simulink model "mariner_simtr"  (R2018b)
settings: Solver=FixedStepAuto  StartTime=0.0  StopTime=600  FixedStep=0.1  RelTol=1e-3
libraries: neural x211, simulink x2
(part 2 of 10)

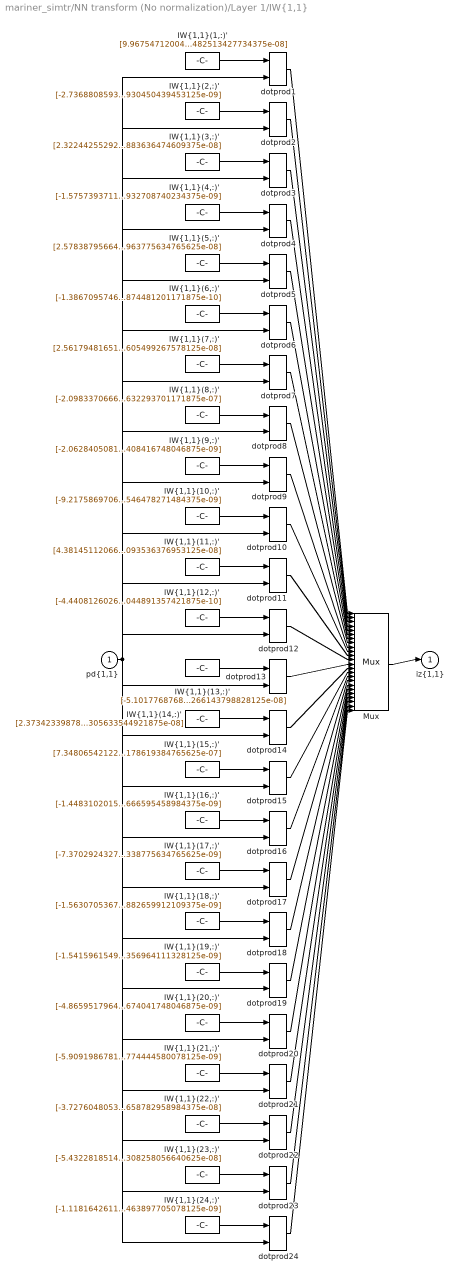
== system mariner_simtr/NN transform (No normalization)/Layer 1/IW{1,1} ==
  "pd{1,1}" : Inport  PortDimensions=7
      mask Display: e = 0.06;c1 = [120 230 180]/255;c2 = ([120 230 180]+0)/(256+128);c3 = ([120 230 180]+128)/(256+128);patch([0 1 1 0],[0 0 1 1],c1);patch([0 1 1 1-e 1-e 0+e],[0 0 1 1-e 0+e 0+e],c2);patch([0 0 1 1-e 0+e 0+e],[0 1 1 1-e 1-e 0+e],c3);plot([0 1 1 0 0],[0 0 1 1 0]);
  "IW{1,1}(1,:)'" : Constant  Value=[9.96754712004838051999594400747091438308444821814191527664661407470703125e-10;-4.23539616837629799060249528863675294587665121071040630340576171875e-08;1.955485657944718495509006986853017817651334553374908864498138427734375e-08;-4.070098816021972745819758874620541977407128797494806349277496337890625e-08;4.66661762648838560338676137331619109271940715188975445926189422607421875e-09;-4.813604277413395185011998032853508533435160643421113491058349609375e-08;-3.648399644882457702946610181814202089611853807582519948482513427734375e-08]
      mask Display: e = 0.06;c1 = [120 150 230]/255;c2 = ([120 150 230]+0)/383;c3 = ([120 150 230]+128)/383;patch([0 1 1 0],[0 0 1 1],c1);patch([0 1 1 1-e 1-e 0+e],[0 0 1 1-e 0+e 0+e],c2);patch([0 0 1 1-e 0+e 0+e],[0 1 1 1-e 1-e 0+e],c3);plot([0 1 1 0 0],[0 0 1 1 0]);disp('Weights');
  "IW{1,1}(10,:)'" : Constant  Value=[-9.21758697067975692512585843448047473458473177743144333362579345703125e-09;1.5109007388292643668241629927896652052510262365103699266910552978515625e-08;-2.8593879081023034796134684831607486454885247439960949122905731201171875e-08;7.24476771790234500451820988799027378757244832740980200469493865966796875e-09;-2.390110051996968584293398892536008926157364840037189424037933349609375e-08;1.2024606259677698783971109926433686043711901447750278748571872711181640625e-09;-6.3639012808772434761134367798250666137249709208845160901546478271484375e-09]
      mask Display: e = 0.06;c1 = [120 150 230]/255;c2 = ([120 150 230]+0)/383;c3 = ([120 150 230]+128)/383;patch([0 1 1 0],[0 0 1 1],c1);patch([0 1 1 1-e 1-e 0+e],[0 0 1 1-e 0+e 0+e],c2);patch([0 0 1 1-e 0+e 0+e],[0 1 1 1-e 1-e 0+e],c3);plot([0 1 1 0 0],[0 0 1 1 0]);disp('Weights');
  "IW{1,1}(11,:)'" : Constant  Value=[4.38145112066941093156313009928108821722236854157017660327255725860595703125e-10;-2.3609184555780799633161487374559406315910337070818059146404266357421875e-08;1.08683559136344472219348574111054406277077077902504242956638336181640625e-08;-2.2688420071581493037842736592256398520106586147448979318141937255859375e-08;2.577333665822960669212732294909400099225393887536483816802501678466796875e-09;-2.6827945833227834960700084582750635231462865704088471829891204833984375e-08;-2.0338792630435224968121508200454006232149595234659500420093536376953125e-08]
      mask Display: e = 0.06;c1 = [120 150 230]/255;c2 = ([120 150 230]+0)/383;c3 = ([120 150 230]+128)/383;patch([0 1 1 0],[0 0 1 1],c1);patch([0 1 1 1-e 1-e 0+e],[0 0 1 1-e 0+e 0+e],c2);patch([0 0 1 1-e 0+e 0+e],[0 1 1 1-e 1-e 0+e],c3);plot([0 1 1 0 0],[0 0 1 1 0]);disp('Weights');
  "IW{1,1}(12,:)'" : Constant  Value=[-4.44081260262457014744597405086871944046578164488892070949077606201171875e-09;3.18447157678982755093461472391258570979744035867042839527130126953125e-08;-3.32801187487933600657970581969402612543262875988148152828216552734375e-08;2.014363404465310276539939909716536714512358230422250926494598388671875e-08;-2.7009658392937414758657856746378034262789924468961544334888458251953125e-08;1.04114761496777040929841848184052299775004257753607816994190216064453125e-08;-8.5873020309611764853519627507631717389102732340688817203044891357421875e-10]
      mask Display: e = 0.06;c1 = [120 150 230]/255;c2 = ([120 150 230]+0)/383;c3 = ([120 150 230]+128)/383;patch([0 1 1 0],[0 0 1 1],c1);patch([0 1 1 1-e 1-e 0+e],[0 0 1 1-e 0+e 0+e],c2);patch([0 0 1 1-e 0+e 0+e],[0 1 1 1-e 1-e 0+e],c3);plot([0 1 1 0 0],[0 0 1 1 0]);disp('Weights');
  "IW{1,1}(13,:)'" : Constant  Value=[-5.1017768768232909158035349832249760737568067270331084728240966796875e-09;1.099732326060325747775131880433485687120764850988052785396575927734375e-07;-9.6376903694374034393577859759771886416501729399897158145904541015625e-08;7.702898533754286069518703826408678736470392323099076747894287109375e-08;-7.235783348817856666161077612564600514133417163975536823272705078125e-08;5.267928186779311432795554876427901458413316504447720944881439208984375e-08;1.7345726966175917324916222928173070716439951866050250828266143798828125e-08]
      mask Display: e = 0.06;c1 = [120 150 230]/255;c2 = ([120 150 230]+0)/383;c3 = ([120 150 230]+128)/383;patch([0 1 1 0],[0 0 1 1],c1);patch([0 1 1 1-e 1-e 0+e],[0 0 1 1-e 0+e 0+e],c2);patch([0 0 1 1-e 0+e 0+e],[0 1 1 1-e 1-e 0+e],c3);plot([0 1 1 0 0],[0 0 1 1 0]);disp('Weights');
  "IW{1,1}(14,:)'" : Constant  Value=[2.37342339878500993051951858492203129014086471215705387294292449951171875e-09;-6.9409118276585255820877663930634771105587788042612373828887939453125e-08;3.232449834280652108462386488431372644214434330933727324008941650390625e-08;-6.66896830743175840225939860449189122704183319001458585262298583984375e-08;7.8615207967289628717666078220292769085375539361848495900630950927734375e-09;-7.8902832936415914953927710530356964824250098899938166141510009765625e-08;-5.975529031343248632389994305647018535410097683779895305633544921875e-08]
      mask Display: e = 0.06;c1 = [120 150 230]/255;c2 = ([120 150 230]+0)/383;c3 = ([120 150 230]+128)/383;patch([0 1 1 0],[0 0 1 1],c1);patch([0 1 1 1-e 1-e 0+e],[0 0 1 1-e 0+e 0+e],c2);patch([0 0 1 1-e 0+e 0+e],[0 1 1 1-e 1-e 0+e],c3);plot([0 1 1 0 0],[0 0 1 1 0]);disp('Weights');
  "IW{1,1}(15,:)'" : Constant  Value=[7.3480654212243858235158316407308054518665585419512353837490081787109375e-09;-1.37910872201280553869879772453665989218052345677278935909271240234375e-07;6.6144410053191093139834965709822345303336987853981554508209228515625e-08;-1.3245204146490021739396747597894421488717853208072483539581298828125e-07;1.708616089860501443057811429664105684622654734994284808635711669921875e-08;-1.56945855317767068446145844844152872354925420950166881084442138671875e-07;-1.18534841031160093440845193502042320687905885279178619384765625e-07]
      mask Display: e = 0.06;c1 = [120 150 230]/255;c2 = ([120 150 230]+0)/383;c3 = ([120 150 230]+128)/383;patch([0 1 1 0],[0 0 1 1],c1);patch([0 1 1 1-e 1-e 0+e],[0 0 1 1-e 0+e 0+e],c2);patch([0 0 1 1-e 0+e 0+e],[0 1 1 1-e 1-e 0+e],c3);plot([0 1 1 0 0],[0 0 1 1 0]);disp('Weights');
  "IW{1,1}(16,:)'" : Constant  Value=[-1.4483102015300659619008766631326722007511165202231495641171932220458984375e-09;3.053887482089307960456361803851244030028055931325070559978485107421875e-08;-2.68218652011502346177757743518610400457191644818522036075592041015625e-08;2.13794257743043844947837517876665369698230279027484357357025146484375e-08;-2.014676439457038581716768858853594537094977567903697490692138671875e-08;1.460163542807002359793662449836959549287485060631297528743743896484375e-08;4.7860605580468106034501928731060560462395869762985967099666595458984375e-09]
      mask Display: e = 0.06;c1 = [120 150 230]/255;c2 = ([120 150 230]+0)/383;c3 = ([120 150 230]+128)/383;patch([0 1 1 0],[0 0 1 1],c1);patch([0 1 1 1-e 1-e 0+e],[0 0 1 1-e 0+e 0+e],c2);patch([0 0 1 1-e 0+e 0+e],[0 1 1 1-e 1-e 0+e],c3);plot([0 1 1 0 0],[0 0 1 1 0]);disp('Weights');
  "IW{1,1}(17,:)'" : Constant  Value=[-7.37029243278886431384240804387010526088630513186217285692691802978515625e-09;5.13920169010480328451178516115105399109097561449743807315826416015625e-08;-5.406989574538547646120274282367790252834538478055037558078765869140625e-08;3.244029838149221145765052523417260044169552202220074832439422607421875e-08;-4.391888903266115245392352023530435634057766947080381214618682861328125e-08;1.6673505568151500479441917755389634958618216842296533286571502685546875e-08;-1.572529870117332454563925412207615883719569183085695840418338775634765625e-09]
      mask Display: e = 0.06;c1 = [120 150 230]/255;c2 = ([120 150 230]+0)/383;c3 = ([120 150 230]+128)/383;patch([0 1 1 0],[0 0 1 1],c1);patch([0 1 1 1-e 1-e 0+e],[0 0 1 1-e 0+e 0+e],c2);patch([0 0 1 1-e 0+e 0+e],[0 1 1 1-e 1-e 0+e],c3);plot([0 1 1 0 0],[0 0 1 1 0]);disp('Weights');
  "IW{1,1}(18,:)'" : Constant  Value=[-1.5630705367480064101360989086732244945920911050052382051944732666015625e-08;1.2844123921892863398315043181596717403181173722259700298309326171875e-07;-1.30133673686686352043631186188588078067596143228001892566680908203125e-07;8.200088059824167129705668223549341888656272203661501407623291015625e-08;-1.05215545994692440098363457774699458724398937192745506763458251953125e-07;4.33666531310121004011057764537806491489391191862523555755615234375e-08;-1.28883019475470923089079378922282292929679670123732648789882659912109375e-09]
      mask Display: e = 0.06;c1 = [120 150 230]/255;c2 = ([120 150 230]+0)/383;c3 = ([120 150 230]+128)/383;patch([0 1 1 0],[0 0 1 1],c1);patch([0 1 1 1-e 1-e 0+e],[0 0 1 1-e 0+e 0+e],c2);patch([0 0 1 1-e 0+e 0+e],[0 1 1 1-e 1-e 0+e],c3);plot([0 1 1 0 0],[0 0 1 1 0]);disp('Weights');
  "IW{1,1}(19,:)'" : Constant  Value=[-1.5415961549154450456600809560921312713066555488694575615227222442626953125e-09;3.3170310091952161113895030698783816802688306779600679874420166015625e-08;-2.907377317587945963731183257432177935442041416536085307598114013671875e-08;2.3233161307144997984342005910469997065348479736712761223316192626953125e-08;-2.1829287747494461351506497641915272023283023372641764581203460693359375e-08;1.5888289744811928436986789791272867145011105094454251229763031005859375e-08;5.23023291522121942520652288118043760078990089823491871356964111328125e-09]
      mask Display: e = 0.06;c1 = [120 150 230]/255;c2 = ([120 150 230]+0)/383;c3 = ([120 150 230]+128)/383;patch([0 1 1 0],[0 0 1 1],c1);patch([0 1 1 1-e 1-e 0+e],[0 0 1 1-e 0+e 0+e],c2);patch([0 0 1 1-e 0+e 0+e],[0 1 1 1-e 1-e 0+e],c3);plot([0 1 1 0 0],[0 0 1 1 0]);disp('Weights');
  "IW{1,1}(2,:)'" : Constant  Value=[-2.736880859346069335748875792926025629636654912246740423142910003662109375e-09;5.902694971324982067598831770964540321955382751184515655040740966796875e-08;-5.1728078424699451181702843267917746317152705159969627857208251953125e-08;4.134227531808641390325789505451326011353785361279733479022979736328125e-08;-3.88368911181434744954370599269444230827730279997922480106353759765625e-08;2.827394876174494392768362098673773363799455182743258774280548095703125e-08;9.309327476142742333364672670421857691991363026318140327930450439453125e-09]
      mask Display: e = 0.06;c1 = [120 150 230]/255;c2 = ([120 150 230]+0)/383;c3 = ([120 150 230]+128)/383;patch([0 1 1 0],[0 0 1 1],c1);patch([0 1 1 1-e 1-e 0+e],[0 0 1 1-e 0+e 0+e],c2);patch([0 0 1 1-e 0+e 0+e],[0 1 1 1-e 1-e 0+e],c3);plot([0 1 1 0 0],[0 0 1 1 0]);disp('Weights');
  "IW{1,1}(20,:)'" : Constant  Value=[-4.86595179647605248405393629459493587408047687858925200998783111572265625e-09;3.26657871565783989586747465029559212013055002898909151554107666015625e-08;-3.469893074219905699171392628003818270343572294223122298717498779296875e-08;2.0560448490772478499383980519131520647846400606795214116573333740234375e-08;-2.82148079239193913611238287604543462094852657173760235309600830078125e-08;1.04905239479849043770109628362537101953222418160294182598590850830078125e-08;-1.1689321922241270052697945862167638875206421289476566016674041748046875e-09]
      mask Display: e = 0.06;c1 = [120 150 230]/255;c2 = ([120 150 230]+0)/383;c3 = ([120 150 230]+128)/383;patch([0 1 1 0],[0 0 1 1],c1);patch([0 1 1 1-e 1-e 0+e],[0 0 1 1-e 0+e 0+e],c2);patch([0 0 1 1-e 0+e 0+e],[0 1 1 1-e 1-e 0+e],c3);plot([0 1 1 0 0],[0 0 1 1 0]);disp('Weights');
  "IW{1,1}(21,:)'" : Constant  Value=[-5.90919867818142536771689580263160201933914095207001082599163055419921875e-09;4.23596922702509948620164660464115780058591553824953734874725341796875e-08;-4.427960655273123418020127391690754503628113525337539613246917724609375e-08;2.6791635390820279313359056176657713166378016467206180095672607421875e-08;-3.593839528671613701771831816782210022864774146000854671001434326171875e-08;1.38421177630135737742344206207580070699947327739209868013858795166015625e-08;-1.1607068937858028159101323080470979931533292983658611774444580078125e-09]
      mask Display: e = 0.06;c1 = [120 150 230]/255;c2 = ([120 150 230]+0)/383;c3 = ([120 150 230]+128)/383;patch([0 1 1 0],[0 0 1 1],c1);patch([0 1 1 1-e 1-e 0+e],[0 0 1 1-e 0+e 0+e],c2);patch([0 0 1 1-e 0+e 0+e],[0 1 1 1-e 1-e 0+e],c3);plot([0 1 1 0 0],[0 0 1 1 0]);disp('Weights');
  "IW{1,1}(22,:)'" : Constant  Value=[-3.727604805384169344832192877388366003543751503457315266132354736328125e-08;1.172724790951451694969578996678716276136356100323610007762908935546875e-07;-1.6014903040348191092204113532282416798580015893094241619110107421875e-07;6.73183958318854417049261255022452044016745276167057454586029052734375e-08;-1.31550756612420119907568287660748485023987086606211960315704345703125e-07;2.778369009628760810329470829806164378084076815866865217685699462890625e-08;-2.029709699747728526551498301998266438062046290724538266658782958984375e-08]
      mask Display: e = 0.06;c1 = [120 150 230]/255;c2 = ([120 150 230]+0)/383;c3 = ([120 150 230]+128)/383;patch([0 1 1 0],[0 0 1 1],c1);patch([0 1 1 1-e 1-e 0+e],[0 0 1 1-e 0+e 0+e],c2);patch([0 0 1 1-e 0+e 0+e],[0 1 1 1-e 1-e 0+e],c3);plot([0 1 1 0 0],[0 0 1 1 0]);disp('Weights');
  "IW{1,1}(23,:)'" : Constant  Value=[-5.43228185145061583705953608849741065522920280272956006228923797607421875e-09;1.170978675560962556496971101634152478965233967755921185016632080078125e-07;-1.026199558971175130461586113249372598232866948819719254970550537109375e-07;8.2020122441372280621760672107700695931953305262140929698944091796875e-08;-7.70466698024706418528796572457728597527193414862267673015594482421875e-08;5.609342392485284586896892764472377646001177708967588841915130615234375e-08;1.846762772031701079541643668348316342786574750789441168308258056640625e-08]
      mask Display: e = 0.06;c1 = [120 150 230]/255;c2 = ([120 150 230]+0)/383;c3 = ([120 150 230]+128)/383;patch([0 1 1 0],[0 0 1 1],c1);patch([0 1 1 1-e 1-e 0+e],[0 0 1 1-e 0+e 0+e],c2);patch([0 0 1 1-e 0+e 0+e],[0 1 1 1-e 1-e 0+e],c3);plot([0 1 1 0 0],[0 0 1 1 0]);disp('Weights');
  "IW{1,1}(24,:)'" : Constant  Value=[-1.11816426113187927785879471659531703142675951312412507832050323486328125e-08;9.179529262955325056978187099610000387883701478131115436553955078125e-08;-9.30252272128869384096500928793549434203669079579412937164306640625e-08;5.858745564967901846581630202932811091187659258139319717884063720703125e-08;-7.52286172919048964737097177912783507736094179563224315643310546875e-08;3.096918421804722152496116530269454347745750055764801800251007080078125e-08;-1.002465361068514032997859634324840094610209462189231999218463897705078125e-09]
      mask Display: e = 0.06;c1 = [120 150 230]/255;c2 = ([120 150 230]+0)/383;c3 = ([120 150 230]+128)/383;patch([0 1 1 0],[0 0 1 1],c1);patch([0 1 1 1-e 1-e 0+e],[0 0 1 1-e 0+e 0+e],c2);patch([0 0 1 1-e 0+e 0+e],[0 1 1 1-e 1-e 0+e],c3);plot([0 1 1 0 0],[0 0 1 1 0]);disp('Weights');
  "IW{1,1}(3,:)'" : Constant  Value=[2.3224425529203732312677545030106529555524730312754400074481964111328125e-09;-6.79293542914116131004281622096652171194364200346171855926513671875e-08;3.16325922238083046083605078153955236786032401141710579395294189453125e-08;-6.5269718938136910214959057578709700209174116025678813457489013671875e-08;7.69150849643806513870867322228697116059947802568785846233367919921875e-09;-7.72232186310361172496818655923422891618201902019791305065155029296875e-08;-5.84843975722607335487583809195688555604419889277778565883636474609375e-08]
      mask Display: e = 0.06;c1 = [120 150 230]/255;c2 = ([120 150 230]+0)/383;c3 = ([120 150 230]+128)/383;patch([0 1 1 0],[0 0 1 1],c1);patch([0 1 1 1-e 1-e 0+e],[0 0 1 1-e 0+e 0+e],c2);patch([0 0 1 1-e 0+e 0+e],[0 1 1 1-e 1-e 0+e],c3);plot([0 1 1 0 0],[0 0 1 1 0]);disp('Weights');
  "IW{1,1}(4,:)'" : Constant  Value=[-1.5757393711212239489573953290200980514867978854454122483730316162109375e-09;3.398105935002767075160871163529152649829256915836594998836517333984375e-08;-2.97794683945180708540138359886884078520097318687476217746734619140625e-08;2.380147629323289543301717867233857628406212825211696326732635498046875e-08;-2.2358315984684428928152047887090159150602630688808858394622802734375e-08;1.627722399093271681704852052972876119696366004063747823238372802734375e-08;5.3590863849978235579479203163320855107798479366465471684932708740234375e-09]
      mask Display: e = 0.06;c1 = [120 150 230]/255;c2 = ([120 150 230]+0)/383;c3 = ([120 150 230]+128)/383;patch([0 1 1 0],[0 0 1 1],c1);patch([0 1 1 1-e 1-e 0+e],[0 0 1 1-e 0+e 0+e],c2);patch([0 0 1 1-e 0+e 0+e],[0 1 1 1-e 1-e 0+e],c3);plot([0 1 1 0 0],[0 0 1 1 0]);disp('Weights');
  "IW{1,1}(5,:)'" : Constant  Value=[2.578387956646821386262262190930232008678757438246975652873516082763671875e-10;-1.39061626338902988860742851624785476616352752898819744586944580078125e-08;6.40125093731916103556093254091374777914325022720731794834136962890625e-09;-1.33639767245069021187178214828648881162820316603756509721279144287109375e-08;1.5179028736585700792937570096133824415485236158929183147847652435302734375e-09;-1.580227044658806774721533238044213209860799906891770660877227783203125e-08;-1.1980281539188823830406369443969671895189321730867959558963775634765625e-08]
      mask Display: e = 0.06;c1 = [120 150 230]/255;c2 = ([120 150 230]+0)/383;c3 = ([120 150 230]+128)/383;patch([0 1 1 0],[0 0 1 1],c1);patch([0 1 1 1-e 1-e 0+e],[0 0 1 1-e 0+e 0+e],c2);patch([0 0 1 1-e 0+e 0+e],[0 1 1 1-e 1-e 0+e],c3);plot([0 1 1 0 0],[0 0 1 1 0]);disp('Weights');
  "IW{1,1}(6,:)'" : Constant  Value=[-1.3867095746777479392709234935266750243787470253664650954306125640869140625e-09;1.14066147117358784886158936007494180131516259280033409595489501953125e-08;-1.15553235223709413058554965644635081911673069043899886310100555419921875e-08;7.279280159413825905859356051562369938068286501220427453517913818359375e-09;-9.3463069187052717682138907391749260700208878915873356163501739501953125e-09;3.8464198353759935298473327945807664907107437102240510284900665283203125e-09;-1.273779272363968995991060355698720578387916901874632458202540874481201171875e-10]
      mask Display: e = 0.06;c1 = [120 150 230]/255;c2 = ([120 150 230]+0)/383;c3 = ([120 150 230]+128)/383;patch([0 1 1 0],[0 0 1 1],c1);patch([0 1 1 1-e 1-e 0+e],[0 0 1 1-e 0+e 0+e],c2);patch([0 0 1 1-e 0+e 0+e],[0 1 1 1-e 1-e 0+e],c3);plot([0 1 1 0 0],[0 0 1 1 0]);disp('Weights');
  "IW{1,1}(7,:)'" : Constant  Value=[2.561794816514778783262103480067826966060096083310781978070735931396484375e-10;-1.380210707037911175766410685865348551004672117414884269237518310546875e-08;6.35276019390252450627447865227903633922323933802545070648193359375e-09;-1.32640168703112810743202282562878957516971922814263962209224700927734375e-08;1.5058978574009581085089311055656875748542944393193465657532215118408203125e-09;-1.5685037309467738701051155625516841940481072015245445072650909423828125e-08;-1.1891651183705094023693456359476450234780031678383238613605499267578125e-08]
      mask Display: e = 0.06;c1 = [120 150 230]/255;c2 = ([120 150 230]+0)/383;c3 = ([120 150 230]+128)/383;patch([0 1 1 0],[0 0 1 1],c1);patch([0 1 1 1-e 1-e 0+e],[0 0 1 1-e 0+e 0+e],c2);patch([0 0 1 1-e 0+e 0+e],[0 1 1 1-e 1-e 0+e],c3);plot([0 1 1 0 0],[0 0 1 1 0]);disp('Weights');
  "IW{1,1}(8,:)'" : Constant  Value=[-2.098337066680637515982030296400086266661588751958333887159824371337890625e-09;-2.012744499847773860113221526535465244478473323397338390350341796875e-07;9.13914835017614789813164230015962719022581950412131845951080322265625e-08;-1.9346416131584142649138167123490372745209242566488683223724365234375e-07;2.1007094255205750548163318321658044052213654140359722077846527099609375e-08;-2.2860633849821883474575626334079903045903847669251263141632080078125e-07;-1.7352583730535906258679135043265784332788825850002467632293701171875e-07]
      mask Display: e = 0.06;c1 = [120 150 230]/255;c2 = ([120 150 230]+0)/383;c3 = ([120 150 230]+128)/383;patch([0 1 1 0],[0 0 1 1],c1);patch([0 1 1 1-e 1-e 0+e],[0 0 1 1-e 0+e 0+e],c2);patch([0 0 1 1-e 0+e 0+e],[0 1 1 1-e 1-e 0+e],c3);plot([0 1 1 0 0],[0 0 1 1 0]);disp('Weights');
  "IW{1,1}(9,:)'" : Constant  Value=[-2.0628405081894719967934079935499569469214975470094941556453704833984375e-08;1.60728119705768779211727524149078139004132026457227766513824462890625e-07;-1.64788974609277832402074435470817892479544752859510481357574462890625e-07;1.0225529152247166173080451627430687011610643821768462657928466796875e-07;-1.33437713545835176052803123895873493864883130299858748912811279296875e-07;5.35971620388351293285411906970605588895750770461745560169219970703125e-08;-2.757314565971735213566048015225266876182530495498212985694408416748046875e-09]
      mask Display: e = 0.06;c1 = [120 150 230]/255;c2 = ([120 150 230]+0)/383;c3 = ([120 150 230]+128)/383;patch([0 1 1 0],[0 0 1 1],c1);patch([0 1 1 1-e 1-e 0+e],[0 0 1 1-e 0+e 0+e],c2);patch([0 0 1 1-e 0+e 0+e],[0 1 1 1-e 1-e 0+e],c3);plot([0 1 1 0 0],[0 0 1 1 0]);disp('Weights');
  Mux : Mux  Inputs=24
      mask Display: e = 0.06;c1 = [120 150 230]/255;c2 = ([120 150 230]+0)/383;c3 = ([120 150 230]+128)/383;patch([0 1 1 0],[0 0 1 1],c1);patch([0 1 1 1-e 1-e 0+e],[0 0 1 1-e 0+e 0+e],c2);patch([0 0 1 1-e 0+e 0+e],[0 1 1 1-e 1-e 0+e],c3);plot([0 1 1 0 0],[0 0 1 1 0]);disp('Mux');
  dotprod{1..24} (24 alike) : neural/Weight Functions/dotprod
  "iz{1,1}" : Outport
      mask Display: e = 0.06;c1 = [120 230 180]/255;c2 = ([120 230 180]+0)/(256+128);c3 = ([120 230 180]+128)/(256+128);patch([0 1 1 0],[0 0 1 1],c1);patch([0 1 1 1-e 1-e 0+e],[0 0 1 1-e 0+e 0+e],c2);patch([0 0 1 1-e 0+e 0+e],[0 1 1 1-e 1-e 0+e],c3);plot([0 1 1 0 0],[0 0 1 1 0]);
  wires:
  Mux/1 -> "iz{1,1}"/1
  dotprod24/1 -> Mux/24
  "IW{1,1}(24,:)'"/1 -> dotprod24/1
  dotprod23/1 -> Mux/23
  "IW{1,1}(23,:)'"/1 -> dotprod23/1
  dotprod22/1 -> Mux/22
  "IW{1,1}(22,:)'"/1 -> dotprod22/1
  dotprod21/1 -> Mux/21
  "IW{1,1}(21,:)'"/1 -> dotprod21/1
  dotprod20/1 -> Mux/20
  "IW{1,1}(20,:)'"/1 -> dotprod20/1
  dotprod19/1 -> Mux/19
  "IW{1,1}(19,:)'"/1 -> dotprod19/1
  dotprod18/1 -> Mux/18
  "IW{1,1}(18,:)'"/1 -> dotprod18/1
  dotprod17/1 -> Mux/17
  "IW{1,1}(17,:)'"/1 -> dotprod17/1
  dotprod16/1 -> Mux/16
  "IW{1,1}(16,:)'"/1 -> dotprod16/1
  dotprod15/1 -> Mux/15
  "IW{1,1}(15,:)'"/1 -> dotprod15/1
  dotprod14/1 -> Mux/14
  "IW{1,1}(14,:)'"/1 -> dotprod14/1
  dotprod13/1 -> Mux/13
  "IW{1,1}(13,:)'"/1 -> dotprod13/1
  dotprod12/1 -> Mux/12
  "IW{1,1}(12,:)'"/1 -> dotprod12/1
  dotprod11/1 -> Mux/11
  "IW{1,1}(11,:)'"/1 -> dotprod11/1
  dotprod10/1 -> Mux/10
  "IW{1,1}(10,:)'"/1 -> dotprod10/1
  dotprod9/1 -> Mux/9
  "IW{1,1}(9,:)'"/1 -> dotprod9/1
  dotprod8/1 -> Mux/8
  "IW{1,1}(8,:)'"/1 -> dotprod8/1
  dotprod7/1 -> Mux/7
  "IW{1,1}(7,:)'"/1 -> dotprod7/1
  dotprod6/1 -> Mux/6
  "IW{1,1}(6,:)'"/1 -> dotprod6/1
  dotprod5/1 -> Mux/5
  "IW{1,1}(5,:)'"/1 -> dotprod5/1
  dotprod4/1 -> Mux/4
  "IW{1,1}(4,:)'"/1 -> dotprod4/1
  dotprod3/1 -> Mux/3
  "IW{1,1}(3,:)'"/1 -> dotprod3/1
  dotprod2/1 -> Mux/2
  "IW{1,1}(2,:)'"/1 -> dotprod2/1
  dotprod1/1 -> Mux/1
  "pd{1,1}"/1 -> dotprod24/2, dotprod23/2, dotprod22/2, dotprod21/2, dotprod20/2, dotprod19/2, dotprod18/2, dotprod17/2, dotprod16/2, dotprod15/2, dotprod14/2, dotprod13/2, dotprod12/2, dotprod11/2, dotprod10/2, dotprod9/2, dotprod8/2, dotprod7/2, dotprod6/2, dotprod5/2, dotprod4/2, dotprod3/2, dotprod2/2, dotprod1/2
  "IW{1,1}(1,:)'"/1 -> dotprod1/1

== system mariner_simtr/NN transform (No normalization)/Layer 2/Delays 1 ==
  "p{2}" : Inport  PortDimensions=24
      mask Display: e = 0.06;c1 = [120 230 180]/255;c2 = ([120 230 180]+0)/(256+128);c3 = ([120 230 180]+128)/(256+128);patch([0 1 1 0],[0 0 1 1],c1);patch([0 1 1 1-e 1-e 0+e],[0 0 1 1-e 0+e 0+e],c2);patch([0 0 1 1-e 0+e 0+e],[0 1 1 1-e 1-e 0+e],c3);plot([0 1 1 0 0],[0 0 1 1 0]);
  mux : Mux  Inputs=1
      mask Display: e = 0.06;c1 = [120 150 230]/255;c2 = ([120 150 230]+0)/383;c3 = ([120 150 230]+128)/383;patch([0 1 1 0],[0 0 1 1],c1);patch([0 1 1 1-e 1-e 0+e],[0 0 1 1-e 0+e 0+e],c2);patch([0 0 1 1-e 0+e 0+e],[0 1 1 1-e 1-e 0+e],c3);plot([0 1 1 0 0],[0 0 1 1 0]);disp('Mux')
  "pd{2,1}" : Outport
      mask Display: e = 0.06;c1 = [120 230 180]/255;c2 = ([120 230 180]+0)/(256+128);c3 = ([120 230 180]+128)/(256+128);patch([0 1 1 0],[0 0 1 1],c1);patch([0 1 1 1-e 1-e 0+e],[0 0 1 1-e 0+e 0+e],c2);patch([0 0 1 1-e 0+e 0+e],[0 1 1 1-e 1-e 0+e],c3);plot([0 1 1 0 0],[0 0 1 1 0]);
  wires:
  mux/1 -> "pd{2,1}"/1
  "p{2}"/1 -> mux/1
